simulink model "simulink_step"  (R2024a)
settings: Solver=VariableStepAuto  StartTime=0.0  StopTime=10.0  RelTol=1e-3
settings Model: Creator=samuel.rovea  LastModifiedBy=franthiescolly.c
settings RTWCC: GPUComputeCapability=3.5

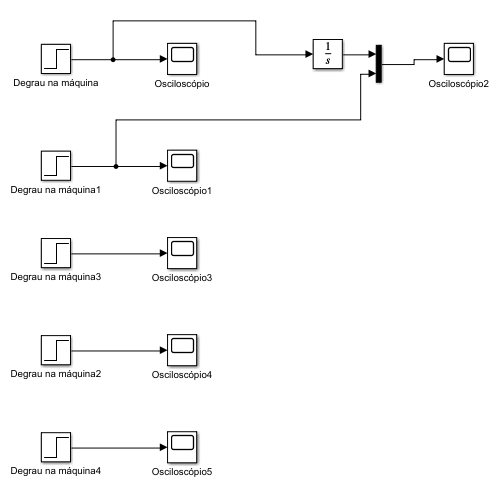
[thumbnail: Simulink's stored preview of the top-level diagram]
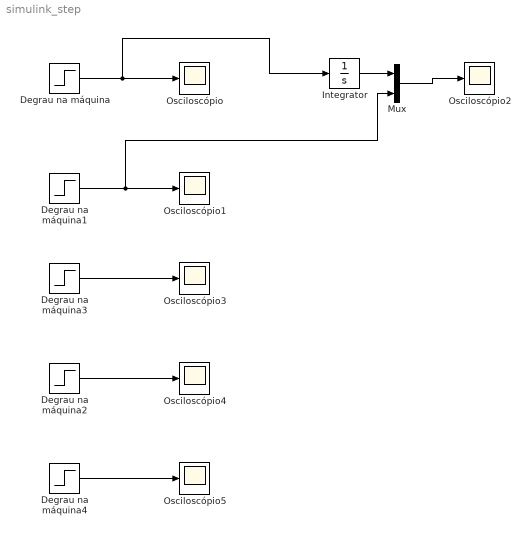
== system simulink_step ==
  Degrau na máquina{,1..4} (5 alike) : Step  After=20  SampleTime=0
  Integrator : Integrator
  Mux : Mux  Inputs=2
  Osciloscópio{,1..5} (6 alike) : Scope
  wires:
  Degrau na máquina/1 -> Integrator/1, Osciloscópio/1
  Degrau na máquina1/1 -> Mux/2, Osciloscópio1/1
  Degrau na máquina3/1 -> Osciloscópio3/1
  Mux/1 -> Osciloscópio2/1
  Integrator/1 -> Mux/1
  Degrau na máquina2/1 -> Osciloscópio4/1
  Degrau na máquina4/1 -> Osciloscópio5/1
